simulink model "TestStructure"  (R2023b)
settings: Solver=FixedStepDiscrete  StartTime=0.0  StopTime=inf  FixedStep=SampleTime  RelTol=1e-3
InitFcn:
  | SampleTime = 0.001;
  | ButtonValue=0;
  | load("BusConfig.mat");
undefined symbols (not defined in the file): DiscIntNeverNeededParam
libraries: slrealtimeethercatlib x219, dspfdesign x28, dspstat3 x23, simulink x21, slpidlib x10, dspswit3 x8, commfilt2 x2, dspsigops x1
(part 4 of 8)

== system TestStructure/InterForceControlTask/AO3/Filter ==
  In : Inport
  Highpass Filter : dspfdesign/Highpass Filter  FilterType=IIR  DesignForMinimumOrder=on  FilterOrder=50  StopbandFrequency=0.015  PassbandFrequency=0.3  StopbandAttenuation=80  PassbandRipple=0.1  SampleRateMode=Specify on dialog  SampleRate=1000  SimulateUsing=Interpreted execution  roundingMode=Floor  coeffsDataTypeStr=fixdt(1,16)
  Highpass Filter1 : dspfdesign/Highpass Filter  FilterType=IIR  DesignForMinimumOrder=on  FilterOrder=50  StopbandFrequency=0.2  PassbandFrequency=0.3  StopbandAttenuation=60  PassbandRipple=1  SampleRateMode=Specify on dialog  SampleRate=1000  SimulateUsing=Code generation  roundingMode=Floor  coeffsDataTypeStr=fixdt(1,16)
  Lowpass Filter : dspfdesign/Lowpass Filter  FilterType=IIR  DesignForMinimumOrder=on  FilterOrder=50  PassbandFrequency=2.3  StopbandFrequency=4.3  PassbandRipple=0.1  StopbandAttenuation=80  SampleRateMode=Specify on dialog  SampleRate=1000  SimulateUsing=Interpreted execution  roundingMode=Floor  coeffsDataTypeStr=fixdt(1,16)
  Lowpass Filter1 : dspfdesign/Lowpass Filter  FilterType=IIR  DesignForMinimumOrder=on  FilterOrder=50  PassbandFrequency=6  StopbandFrequency=8  PassbandRipple=1  StopbandAttenuation=60  SampleRateMode=Specify on dialog  SampleRate=1000  SimulateUsing=Code generation  roundingMode=Floor  coeffsDataTypeStr=fixdt(1,16)
  Out : Outport
  wires:
  Highpass Filter1/1 -> Lowpass Filter1/1
  In/1 -> Highpass Filter/1
  Lowpass Filter/1 -> Out/1
  Highpass Filter/1 -> Lowpass Filter/1

== system TestStructure/InterForceControlTask/AO3/PhaseCorrection ==
  note: Subsystem
  Peaks : Inport
  Clock : Clock
  Constant3 : Constant
  Discrete-Time Integrator : DiscreteIntegrator  ExternalReset=rising  SampleTime=-1  ICPrevOutput=DiscIntNeverNeededParam  ICPrevScaledInput=DiscIntNeverNeededParam
  If : If  IfExpression=u1 == 1
  If Action Subsystem : Subsystem  TreatAsAtomicUnit=on
  If Action Subsystem1 : Subsystem  TreatAsAtomicUnit=on
  MATLAB Function : MATLAB Function  TreatAsAtomicUnit=on
  MATLAB Function1 : MATLAB Function  TreatAsAtomicUnit=on
  Merge : Merge
  Omega : Outport
  Phi_Corrected : Outport  Port=2
  wires:
  Clock/1 -> MATLAB Function1/2(t)
  MATLAB Function1/1(valid_peak) -> If/1
  Peaks/1 -> MATLAB Function1/1(raw_peak)
  If/1 -> If Action Subsystem/Action
  Discrete-Time Integrator/1 -> MATLAB Function/1(t_t_start)
  If/2 -> If Action Subsystem1/Action
  Merge/1 -> Discrete-Time Integrator/2, MATLAB Function/2(u)
  Constant3/1 -> Discrete-Time Integrator/1
  If Action Subsystem1/1(Out1) -> Merge/2
  If Action Subsystem/1(Out1) -> Merge/1
  MATLAB Function/1(Omega) -> Omega/1
  MATLAB Function/2(phi) -> Phi_Corrected/1

== system TestStructure/InterForceControlTask/AO3/Select ==
  P : Inport
  Phi : Inport  Port=2
  q : Inport  Port=3
  Abs : Abs  SaturateOnIntegerOverflow=off
  Add : Sum
  Add1 : Sum
  Bias1 : Bias  SaturateOnIntegerOverflow=off
  Bias2 : Bias  Bias=-0.001  SaturateOnIntegerOverflow=off
  Data Type Conversion : DataTypeConversion  OutDataTypeStr=double  SaturateOnIntegerOverflow=off  RndMeth=Floor
  Edge Detector : dspswit3/Edge Detector
  Gain1 : Gain  Gain=0.6
  Gain2 : Gain  OutDataTypeStr=Inherit: Same as input  ParamDataTypeStr=Inherit: Same as input
  Gain3 : Gain  Gain=0.1
  If : If  NumInputs=2  IfExpression=(u1 >= 10.5)|(u2 <= 1)
  If Action Subsystem : Subsystem  TreatAsAtomicUnit=on
  If Action Subsystem1 : Subsystem  TreatAsAtomicUnit=on
  MATLAB Function1 : MATLAB Function  TreatAsAtomicUnit=on
  Merge : Merge
  Merge1 : Merge
  Moving Average : dspstat3/Moving Average  Method=Sliding window  ForgettingFactorPort=off  SpecifyWindowLength=on  WindowLength=2000  OverlapLength=1999  AllowArbitraryInputLength=off  ForgettingFactor=0.9  SimulateUsing=Code generation
  Moving Average1 : dspstat3/Moving Average  Method=Sliding window  ForgettingFactorPort=off  SpecifyWindowLength=on  WindowLength=2000  OverlapLength=1999  AllowArbitraryInputLength=off  ForgettingFactor=0.9  SimulateUsing=Code generation
  Saturation : Saturate  UpperLimit=inf  LowerLimit=0
  Phi_Out : Outport
  Phase0Event : Outport  Port=2
  wires:
  Bias1/1 -> If Action Subsystem/2(Phase0)
  If Action Subsystem/2(Phase0Event) -> Merge1/2
  If Action Subsystem1/2(Out2) -> Merge1/1
  If Action Subsystem/1(Phi_Out) -> Merge/2
  Add1/1 -> If/2
  Data Type Conversion/1 -> Gain2/1
  Gain3/1 -> Add1/1
  Moving Average1/1 -> Add1/2
  q/1 -> MATLAB Function1/1(u)
  MATLAB Function1/1(y) -> Abs/1
  Abs/1 -> Moving Average1/1, Gain3/1
  Merge1/1 -> Phase0Event/1
  Merge/1 -> Phi_Out/1
  If/2 -> If Action Subsystem/Action
  Add/1 -> If/1
  If/1 -> If Action Subsystem1/Action
  Gain2/1 -> Bias1/1
  Moving Average/1 -> Add/2
  Saturation/1 -> Edge Detector/1
  Edge Detector/1 -> Data Type Conversion/1
  Phi/1 -> If Action Subsystem/1(Phi), Bias2/1
  Bias2/1 -> Saturation/1
  P/1 -> Moving Average/1, Gain1/1
  Gain1/1 -> Add/1
  If Action Subsystem1/1(Out1) -> Merge/1

== system TestStructure/InterForceControlTask/AO3/Subsystem ==
  q : Inport
  f : Inport  Port=2
  Add : Sum  Inputs=++++
  Gain1 : Gain  Gain=1/(2*pi)
  Gain2 : Gain  Gain=1/(2*pi)
  Subsystem : Subsystem
      settings: PortSchema="{\"entries\":[{\"content\":{\"sides\":[{\"content\":{\"connectorIds\":[\"In1\",\"In2\",\"In3\"]},\"type\":\"ConnectorPlacement.EquallySpacedRectSide\",\"uuid\":\"fcadf485-1c54-4f3f-872d-ec2f9b882f19\"},{\"content\":{\"connectorIds\":[\"Out1\",\"Out2\",\"Out3\",\"Out4\"],\"side\":\"RIGHT\"},\"type\":\"ConnectorPlacement.EquallySpacedRectSide\",\"uuid\":\"c1591880-cfe2-422f-a22e-44609bf238b6\"},{\"content\":{\"connectorIds\":[\"In4\"],\"side\":\"TOP\"},\"type\":\"ConnectorPlacement.EquallySpacedRectSide\",\"uuid\":\"5e5eda86-5041-4cab-91db-6a7c0e12be81\"}]},\"type\":\"ConnectorPlacement.EquallySpacedConnector\",\"uuid\":\"19c16159-ed31-430a-9428-452ee8c26aba\"}],\"packageUris\":[\"http://schema.mathworks.com/mf0/Connector/R2020b\"],\"version\":\"1.0\"}"
  Subsystem1 : Subsystem
  Subsystem2 : Subsystem
      settings: PortSchema="{\"entries\":[{\"content\":{\"sides\":[{\"content\":{\"connectorIds\":[\"In1\",\"In2\",\"In3\"]},\"type\":\"ConnectorPlacement.EquallySpacedRectSide\",\"uuid\":\"8ec379b7-ae46-4480-a29c-58696021cca5\"},{\"content\":{\"connectorIds\":[\"Out1\",\"Out2\",\"Out3\"],\"side\":\"RIGHT\"},\"type\":\"ConnectorPlacement.EquallySpacedRectSide\",\"uuid\":\"cda231b2-17f5-4d36-92f5-7ce39ba724b7\"},{\"content\":{\"connectorIds\":[],\"side\":\"TOP\"},\"type\":\"ConnectorPlacement.EquallySpacedRectSide\",\"uuid\":\"4db6421b-b56f-479d-b059-30db4d04c79c\"},{\"content\":{\"connectorIds\":[\"Out4\"],\"side\":\"BOTTOM\"},\"type\":\"ConnectorPlacement.EquallySpacedRectSide\",\"uuid\":\"ff0451e3-8881-4680-9eeb-8c81f572143a\"}]},\"type\":\"ConnectorPlacement.EquallySpacedConnector\",\"uuid\":\"26cfb436-360b-4c37-a6b2-80fa044f0317\"}],\"packageUris\":[\"http://schema.mathworks.com/mf0/Connector/R2020b\"],\"version\":\"1.0\"}"
  Subsystem3 : Subsystem
  Subsystem5 : Subsystem
  x : Outport
  Omega : Outport  Port=2
  Phi : Outport  Port=3
  P : Outport  Port=4
  wires:
  f/1 -> Subsystem/4(f)
  Subsystem/2(Omega) -> Subsystem1/3(Omega), Subsystem3/2(Omega), Subsystem5/3(Omega), Gain1/1
  Subsystem2/4(P) -> P/1
  Subsystem5/1(x) -> Add/4
  Subsystem3/1(x) -> Add/3
  Subsystem2/3(P(t)_Phi) -> Subsystem/3(P(t)_Phi), Subsystem1/2(P(t)_Phi), Subsystem3/3(P(t)_Phi), Subsystem5/2(P(t)_Phi)
  Subsystem1/1(x) -> Add/2
  Subsystem2/2(P(t)_Omega) -> Subsystem/2(P(t)_Omega)
  Subsystem2/1(P(t)_x) -> Subsystem/1(P(t)_x), Subsystem1/1(P(t)_x), Subsystem3/1(P(t)_x), Subsystem5/1(P(t)_x)
  Gain1/1 -> Omega/1
  Subsystem/3(Phi) -> Gain2/1
  Subsystem/1(x) -> Add/1
  Gain2/1 -> Phi/1
  Add/1 -> x/1, Subsystem2/2(X(t))
  q/1 -> Subsystem2/1(T(t))

== system TestStructure/InterForceControlTask/AO3/Subsystem1 ==
  note: Subsystem
  note: ZeroCrossFinder
  q : Inport
  Constant3 : Constant
  Discrete Derivative : simulink/Discrete/Discrete Derivative  gainval=1.0  ICPrevScaledInput=0.0  OutMin=[]  OutMax=[]  OutDataType=fixdt(1, 16)  OutScaling=2^-10  DoSatur=off
  Discrete-Time Integrator : DiscreteIntegrator  ExternalReset=rising  SampleTime=-1  ICPrevOutput=DiscIntNeverNeededParam  ICPrevScaledInput=DiscIntNeverNeededParam
  If : If  IfExpression=u1 == 1
  If Action Subsystem : Subsystem  TreatAsAtomicUnit=on
  If Action Subsystem1 : Subsystem  TreatAsAtomicUnit=on
  If Action Subsystem2 : Subsystem  TreatAsAtomicUnit=on
  If Action Subsystem3 : Subsystem  TreatAsAtomicUnit=on
  If1 : If
  Math Function : Math  Operator=reciprocal
  Memory : Memory
  Merge : Merge
  Merge1 : Merge
  Moving Maximum : dspstat3/Moving Maximum  SpecifyWindowLength=on  WindowLength=3  SimulateUsing=Code generation
  Moving Minimum : dspstat3/Moving Minimum  SpecifyWindowLength=on  WindowLength=3  SimulateUsing=Code generation
  Sign : Signum
  Triggered Subsystem : Subsystem  TreatAsAtomicUnit=on
  f : Outport
  Peak : Outport  Port=2
  wires:
  Discrete Derivative/1 -> Sign/1
  Sign/1 -> If1/1
  If1/1 -> If Action Subsystem2/Action
  If1/2 -> If Action Subsystem3/Action
  If Action Subsystem2/1(Out1) -> Merge1/1
  If Action Subsystem3/1(Out1) -> Merge1/2
  q/1 -> Discrete Derivative/1, Moving Minimum/1, If Action Subsystem2/1(q), Moving Maximum/1, If Action Subsystem3/1(q)
  Moving Minimum/1 -> If Action Subsystem2/2(WindowMin)
  Moving Maximum/1 -> If Action Subsystem3/2(WindowMax)
  Discrete-Time Integrator/1 -> Memory/1
  Merge1/1 -> Peak/1, If/1
  If/2 -> If Action Subsystem1/Action
  Merge/1 -> Triggered Subsystem/Trigger, Discrete-Time Integrator/2
  If/1 -> If Action Subsystem/Action
  Constant3/1 -> Discrete-Time Integrator/1
  If Action Subsystem1/1(Out1) -> Merge/2
  If Action Subsystem/1(Out1) -> Merge/1
  Memory/1 -> Triggered Subsystem/1(In1)
  Math Function/1 -> f/1
  Triggered Subsystem/1(t-t_start) -> Math Function/1

== system TestStructure/InterForceControlTask/DMP/ParamLatch ==
  In1 : Inport
  Enable : EnablePort
  Out1 : Outport
  wires:
  In1/1 -> Out1/1

== system TestStructure/InterForceControlTask/DMP/PhaseTimer ==
  t_now : Inport
  Trigger : TriggerPort  VariantControl=(inherit)
  Add : Sum  Inputs=+-
  UD_tlast : UnitDelay  SampleTime=-1  HasFrameUpgradeWarning=on
  ChunkSize : Outport
  wires:
  UD_tlast/1 -> Add/2
  Add/1 -> ChunkSize/1  "t_prev"
  t_now/1 -> Add/1, UD_tlast/1  "t_now"

== system TestStructure/InterForceControlTask/DMP/Subsystem ==
  ratio : Inport
  trig_in : Inport  Port=2
  t_prev : Inport  Port=3
  T_base_default : Inport  Port=4
  tau : Inport  Port=5
  BaseNormalizedStep : Product  Inputs=*/
  BasePeriodFloor : MinMax  Function=max  Inputs=2
  DelaySamplesFromPrev : MATLAB Function  TreatAsAtomicUnit=on
  EventDelay : MATLAB Function  TreatAsAtomicUnit=on
  Gain1 : Gain  Gain=1/1000
  MinBasePeriod : Constant  Value=0.005
  PhiOmega_DelayRebuild : MATLAB Function  TreatAsAtomicUnit=on
  dt1 : Constant  Value=0.001
  Phase0Event_Delay : Outport
  Phi_Delay : Outport  Port=2
  Omega_Delay : Outport  Port=3
  wires:
  DelaySamplesFromPrev/1(N) -> EventDelay/2(N)
  ratio/1 -> DelaySamplesFromPrev/2(ratio)
  t_prev/1 -> DelaySamplesFromPrev/1(t_prev), BasePeriodFloor/1
  trig_in/1 -> EventDelay/1(trig_in)
  dt1/1 -> DelaySamplesFromPrev/3(dt), BaseNormalizedStep/1, PhiOmega_DelayRebuild/2(dt_sec)
  PhiOmega_DelayRebuild/2(omega_delay) -> Gain1/1
  EventDelay/1(out) -> Phase0Event_Delay/1, PhiOmega_DelayRebuild/1(event_delay)
  PhiOmega_DelayRebuild/1(phi_delay) -> Phi_Delay/1
  tau/1 -> EventDelay/3(tau)
  MinBasePeriod/1 -> BasePeriodFloor/2
  BasePeriodFloor/1 -> BaseNormalizedStep/2
  BaseNormalizedStep/1 -> Omega_Delay/1
  T_base_default/1 -> PhiOmega_DelayRebuild/3(T_base_default)

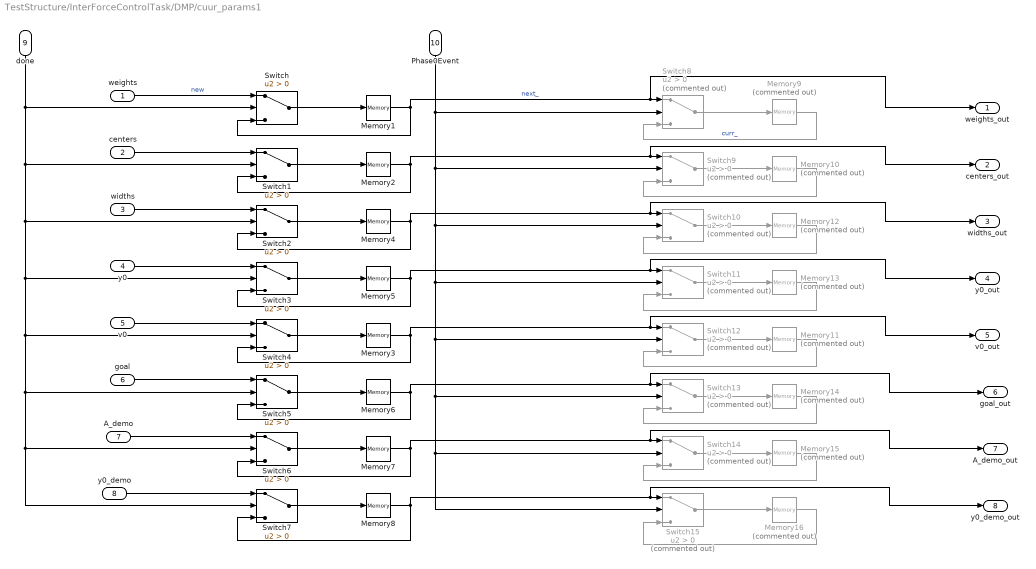
== system TestStructure/InterForceControlTask/DMP/cuur_params1 ==
  weights : Inport
  centers : Inport  Port=2
  widths : Inport  Port=3
  y0 : Inport  Port=4
  v0 : Inport  Port=5
  goal : Inport  Port=6
  A_demo : Inport  Port=7
  y0_demo : Inport  Port=8
  done : Inport  Port=9
  Phase0Event : Inport  Port=10
  Memory{1..2,4,7} (4 alike) : Memory  InitialCondition=1
  Memory{9..10,12,15} (4 alike) : Memory  Commented=on  InitialCondition=1
  Memory{11,13..14,16} (4 alike) : Memory  Commented=on
  Memory{3,5..6,8} (4 alike) : Memory
  Switch{,1..7} (8 alike) : Switch  Criteria=u2 > Threshold  SaturateOnIntegerOverflow=off  InputSameDT=off
  Switch{8..15} (8 alike) : Switch  Commented=on  Criteria=u2 > Threshold  SaturateOnIntegerOverflow=off  InputSameDT=off
  weights_out : Outport
  centers_out : Outport  Port=2
  widths_out : Outport  Port=3
  y0_out : Outport  Port=4
  v0_out : Outport  Port=5
  goal_out : Outport  Port=6
  A_demo_out : Outport  Port=7
  y0_demo_out : Outport  Port=8
  wires:
  Memory10/1 -> Switch9/3
  Switch8/1 -> Memory9/1
  Switch9/1 -> Memory10/1
  Memory1/1 -> Switch8/1, weights_out/1, Switch/3  "next_"
  Switch11/1 -> Memory13/1
  Memory7/1 -> Switch6/3, Switch14/1, A_demo_out/1
  Switch14/1 -> Memory15/1
  Switch10/1 -> Memory12/1
  Switch12/1 -> Memory11/1
  Switch13/1 -> Memory14/1
  Switch15/1 -> Memory16/1
  Phase0Event/1 -> Switch15/2, Switch14/2, Switch13/2, Switch12/2, Switch11/2, Switch10/2, Switch9/2, Switch8/2
  Memory11/1 -> Switch12/3
  Memory6/1 -> Switch5/3, Switch13/1, goal_out/1
  Memory16/1 -> Switch15/3
  Memory15/1 -> Switch14/3
  Memory14/1 -> Switch13/3
  Memory4/1 -> Switch2/3, Switch10/1, widths_out/1
  Memory5/1 -> Switch3/3, Switch11/1, y0_out/1
  Memory12/1 -> Switch10/3
  Memory3/1 -> Switch4/3, Switch12/1, v0_out/1
  Memory2/1 -> Switch1/3, Switch9/1, centers_out/1
  Memory9/1 -> Switch8/3  "curr_"
  Memory13/1 -> Switch11/3
  Memory8/1 -> Switch7/3, Switch15/1, y0_demo_out/1
  weights/1 -> Switch/1  "new"
  centers/1 -> Switch1/1
  widths/1 -> Switch2/1
  y0/1 -> Switch3/1
  v0/1 -> Switch4/1
  goal/1 -> Switch5/1
  A_demo/1 -> Switch6/1
  y0_demo/1 -> Switch7/1
  done/1 -> Switch/2, Switch1/2, Switch2/2, Switch3/2, Switch4/2, Switch5/2, Switch6/2, Switch7/2
  Switch/1 -> Memory1/1
  Switch1/1 -> Memory2/1
  Switch2/1 -> Memory4/1
  Switch3/1 -> Memory5/1
  Switch7/1 -> Memory8/1
  Switch6/1 -> Memory7/1
  Switch5/1 -> Memory6/1
  Switch4/1 -> Memory3/1

== system TestStructure/InterForceControlTask/TorqueController/Filter1 ==
  In : Inport
  Highpass Filter : dspfdesign/Highpass Filter  FilterType=IIR  DesignForMinimumOrder=on  FilterOrder=50  StopbandFrequency=0.015  PassbandFrequency=0.3  StopbandAttenuation=80  PassbandRipple=0.1  SampleRateMode=Specify on dialog  SampleRate=1000  SimulateUsing=Interpreted execution  roundingMode=Floor  coeffsDataTypeStr=fixdt(1,16)
  Highpass Filter1 : dspfdesign/Highpass Filter  FilterType=IIR  DesignForMinimumOrder=on  FilterOrder=50  StopbandFrequency=0.29  PassbandFrequency=0.3  StopbandAttenuation=60  PassbandRipple=1  SampleRateMode=Specify on dialog  SampleRate=1000  SimulateUsing=Code generation  roundingMode=Floor  coeffsDataTypeStr=fixdt(1,16)
  Lowpass Filter : dspfdesign/Lowpass Filter  FilterType=IIR  DesignForMinimumOrder=on  FilterOrder=50  PassbandFrequency=2.3  StopbandFrequency=4.3  PassbandRipple=0.1  StopbandAttenuation=80  SampleRateMode=Specify on dialog  SampleRate=1000  SimulateUsing=Interpreted execution  roundingMode=Floor  coeffsDataTypeStr=fixdt(1,16)
  Lowpass Filter1 : dspfdesign/Lowpass Filter  FilterType=IIR  DesignForMinimumOrder=on  FilterOrder=50  PassbandFrequency=6  StopbandFrequency=8  PassbandRipple=1  StopbandAttenuation=60  SampleRateMode=Specify on dialog  SampleRate=1000  SimulateUsing=Code generation  roundingMode=Floor  coeffsDataTypeStr=fixdt(1,16)
  Out : Outport
  wires:
  Highpass Filter1/1 -> Lowpass Filter1/1
  In/1 -> Highpass Filter1/1
  Lowpass Filter1/1 -> Out/1
  Highpass Filter/1 -> Lowpass Filter/1

== system TestStructure/InterForceControlTask/TorqueController/If Action Subsystem1 ==
  Action Port : ActionPort  ActionPortLabel=if((u1 >= u2))
  ActivityValue : Constant
  activity_gain : Outport
  wires:
  ActivityValue/1 -> activity_gain/1

== system TestStructure/InterForceControlTask/TorqueController/If Action Subsystem_activity_on ==
  Action Port : ActionPort  ActionPortLabel=else
  ActivityValue : Constant  Value=0
  activity_gain : Outport
  wires:
  ActivityValue/1 -> activity_gain/1

== system TestStructure/InterForceControlTask/TorqueController/Subsystem2 ==
  note: ZeroCrossFinder
  q : Inport
  Abs : Abs  Commented=on  SaturateOnIntegerOverflow=off
  Buffer : Buffer  Commented=on  N=30  V=29  OutputFrames=off
  Buffer Function : MATLAB Function  TreatAsAtomicUnit=on
  Constant1 : Constant
  Discrete Derivative : simulink/Discrete/Discrete Derivative  gainval=1.0  ICPrevScaledInput=0.0  OutMin=[]  OutMax=[]  OutDataType=fixdt(1, 16)  OutScaling=2^-10  DoSatur=off
  Function-Call Subsystem : Subsystem  TreatAsAtomicUnit=on
  Function-Call Subsystem1 : Subsystem  TreatAsAtomicUnit=on
  Function-Call Subsystem2 : Subsystem  TreatAsAtomicUnit=on
  Gain : Gain  Gain=0.4
  Gain2 : Gain  Gain=-1
  If Action Subsystem2 : Subsystem  TreatAsAtomicUnit=on
  If Action Subsystem3 : Subsystem  TreatAsAtomicUnit=on
  If1 : If  IfExpression=(u1 > -0.02)&(u1<0.02)
  If2 : If  NumInputs=2  IfExpression=(u1 > u2)  ElseIfExpressions=(u1< -u2)
  MATLAB Function : MATLAB Function  Commented=on  TreatAsAtomicUnit=on
  Merge1 : Merge
  Merge2 : Merge
  Merge3 : Merge  Inputs=3
  Moving Maximum : dspstat3/Moving Maximum  SpecifyWindowLength=on  WindowLength=2000  SimulateUsing=Code generation
  Product : Product
  Switch : Switch  Criteria=u2 > Threshold  SaturateOnIntegerOverflow=off  InputSameDT=off
  Windowed Integrator : commfilt2/Windowed Integrator  Commented=on  integperiod=600  roundingMode=Floor  overflowMode=off  coeffDataTypeStr=Inherit: Same word length as input  coeffMin=[]  coeffMax=[]  coeffLastDataTypeStr=Inherit: Same word length as input  accumDataTypeStr=Inherit: Same as product output  accumLastDataTypeStr=Inherit: Same as product output  outputDataTypeStr=Inherit: Same as accumulator  outputMin=[]  outputMax=[]  outputLastDataTypeStr=Inherit: Same as accumulator
  threadhold : Constant  Value=0.1
  Peak : Outport  OutputWhenDisabled=reset  InitialOutput=[0]
  wires:
  q/1 -> Discrete Derivative/1, Buffer Function/1(u)
  If Action Subsystem3/1(Out1) -> Merge1/2
  If Action Subsystem2/1(Out1) -> Merge1/1
  If1/2 -> If Action Subsystem3/Action
  If1/1 -> If Action Subsystem2/Action
  Discrete Derivative/1 -> If1/1
  Buffer Function/1(y) -> If Action Subsystem2/1(WindowMin)
  If Action Subsystem2/2(Out2) -> Merge2/1
  If Action Subsystem3/2(Out2) -> Merge2/2
  Merge2/1 -> Product/2
  If Action Subsystem2/3(y) -> Product/1
  Function-Call Subsystem/1(Out1) -> Merge3/1  "1"
  Function-Call Subsystem1/1(Out1) -> Merge3/3  "0"
  If2/1 -> Function-Call Subsystem/Action
  If2/3 -> Function-Call Subsystem1/Action
  Function-Call Subsystem2/1(Out1) -> Merge3/2  "-1"
  If2/2 -> Function-Call Subsystem2/Action
  Moving Maximum/1 -> Gain/1
  Gain/1 -> If2/2
  Switch/1 -> If2/1, Moving Maximum/1
  Gain2/1 -> Switch/3
  Constant1/1 -> Switch/2
  Abs/1 -> Windowed Integrator/1
  Windowed Integrator/1 -> MATLAB Function/1(u)
  Product/1 -> Gain2/1, Switch/1, Abs/1
  MATLAB Function/1(y) -> ?
  threadhold/1 -> If Action Subsystem2/2(threadhold)
  Merge3/1 -> Peak/1

== system TestStructure/InterForceControlTask/TorqueController/TorqueManager ==
  activity_enable : Inport
  valid_peak : Inport  Port=2
  target_torque : Inport  Port=3
  MO_drop ? steps : Gain  Gain=0  ParamDataTypeStr=double  OutDataTypeStr=double
  MO_step ramp ? per 5 : Gain  ParamDataTypeStr=double  OutDataTypeStr=double
  activity <= 0 : simulink/Logic and Bit Operations/Compare To Constant  relop=<=  const=0  OutDataTypeStr=boolean
  activity falling edge : Logic  AllPortsSameDT=off  OutDataTypeStr=boolean
  base_gain 0..1 : Saturate  UpperLimit=1  LowerLimit=0  OutDataTypeStr=double
  count + step : Sum  Inputs=++-  OutDataTypeStr=double  AccumDataTypeStr=double
  if activity : simulink/Logic and Bit Operations/Compare To Constant  relop=>  const=0  OutDataTypeStr=boolean
  prev_activity : UnitDelay  SampleTime=-1  HasFrameUpgradeWarning=on
  prev_activity > 0 : simulink/Logic and Bit Operations/Compare To Constant  relop=>  const=0  OutDataTypeStr=boolean
  prev_peak : UnitDelay  SampleTime=-1  HasFrameUpgradeWarning=on
  prev_peak <= 0.5 : simulink/Logic and Bit Operations/Compare To Constant  relop=<=  const=0.5  OutDataTypeStr=boolean
  rising valid step : Logic  Inputs=3  AllPortsSameDT=off  OutDataTypeStr=boolean
  step_count 0..5 : Saturate  UpperLimit=5  LowerLimit=0  OutDataTypeStr=double
  step_count memory : UnitDelay  InitialCondition=0.0  SampleTime=-1  HasFrameUpgradeWarning=on
  torque gate : Product  Inputs=**  OutDataTypeStr=double
  valid_peak > 0.5 : simulink/Logic and Bit Operations/Compare To Constant  relop=>  const=0.5  OutDataTypeStr=boolean
  actual_torque : Outport
  current_gain : Outport  Port=2
  wires:
  valid_peak/1 -> valid_peak > 0.5/1, prev_peak/1
  prev_peak/1 -> prev_peak <= 0.5/1
  valid_peak > 0.5/1 -> rising valid step/1
  prev_peak <= 0.5/1 -> rising valid step/2
  activity_enable/1 -> if activity/1, activity <= 0/1, prev_activity/1
  if activity/1 -> rising valid step/3
  step_count memory/1 -> count + step/1
  rising valid step/1 -> count + step/2
  count + step/1 -> step_count 0..5/1
  MO_step ramp ? per 5/1 -> base_gain 0..1/1
  base_gain 0..1/1 -> current_gain/1, torque gate/2
  target_torque/1 -> torque gate/1
  torque gate/1 -> actual_torque/1
  prev_activity > 0/1 -> activity falling edge/2
  prev_activity/1 -> prev_activity > 0/1
  activity <= 0/1 -> activity falling edge/1
  activity falling edge/1 -> MO_drop ? steps/1
  MO_drop ? steps/1 -> count + step/3
  step_count 0..5/1 -> step_count memory/1, MO_step ramp ? per 5/1

== system TestStructure/InterForceControlTask/TorqueController2/Filter ==
  q : Inport
  Highpass Filter : dspfdesign/Highpass Filter  FilterType=IIR  DesignForMinimumOrder=on  FilterOrder=50  StopbandFrequency=0.015  PassbandFrequency=0.3  StopbandAttenuation=80  PassbandRipple=0.1  SampleRateMode=Specify on dialog  SampleRate=1000  SimulateUsing=Interpreted execution  roundingMode=Floor  coeffsDataTypeStr=fixdt(1,16)
  Highpass Filter1 : dspfdesign/Highpass Filter  FilterType=IIR  DesignForMinimumOrder=on  FilterOrder=50  StopbandFrequency=0.2  PassbandFrequency=0.3  StopbandAttenuation=60  PassbandRipple=1  SampleRateMode=Specify on dialog  SampleRate=1000  SimulateUsing=Code generation  roundingMode=Floor  coeffsDataTypeStr=fixdt(1,16)
  Lowpass Filter : dspfdesign/Lowpass Filter  FilterType=IIR  DesignForMinimumOrder=on  FilterOrder=50  PassbandFrequency=2.3  StopbandFrequency=4.3  PassbandRipple=0.1  StopbandAttenuation=80  SampleRateMode=Specify on dialog  SampleRate=1000  SimulateUsing=Interpreted execution  roundingMode=Floor  coeffsDataTypeStr=fixdt(1,16)
  Lowpass Filter1 : dspfdesign/Lowpass Filter  FilterType=IIR  DesignForMinimumOrder=on  FilterOrder=50  PassbandFrequency=6  StopbandFrequency=8  PassbandRipple=1  StopbandAttenuation=60  SampleRateMode=Specify on dialog  SampleRate=1000  SimulateUsing=Code generation  roundingMode=Floor  coeffsDataTypeStr=fixdt(1,16)
  Out : Outport
  wires:
  Highpass Filter1/1 -> Lowpass Filter1/1
  q/1 -> Highpass Filter/1
  Lowpass Filter/1 -> Out/1
  Highpass Filter/1 -> Lowpass Filter/1

== system TestStructure/InterForceControlTask/TorqueController2/ZeroCrossFinder_Right ==
  note: ZeroCrossFinder
  U : Inport
  Discrete Derivative1 : simulink/Discrete/Discrete Derivative  gainval=1.0  ICPrevScaledInput=0.0  OutMin=[]  OutMax=[]  OutDataType=fixdt(1, 16)  OutScaling=2^-10  DoSatur=off
  If Action Subsystem1 : Subsystem  TreatAsAtomicUnit=on
  If Action Subsystem4 : Subsystem  TreatAsAtomicUnit=on
  If2 : If  IfExpression=(u1 > -0.005)|(u1<0.005)
  Merge2 : Merge
  Moving Minimum1 : dspstat3/Moving Minimum  SpecifyWindowLength=on  WindowLength=3  SimulateUsing=Code generation
  peak_right : Outport
  wires:
  U/1 -> Discrete Derivative1/1, Moving Minimum1/1
  If Action Subsystem1/1(Out1) -> Merge2/1
  If Action Subsystem4/1(Out1) -> Merge2/2
  If2/1 -> If Action Subsystem1/Action
  Moving Minimum1/1 -> If Action Subsystem1/1(WindowMin)
  If2/2 -> If Action Subsystem4/Action
  Discrete Derivative1/1 -> If2/1
  Merge2/1 -> peak_right/1

== system TestStructure/InterForceControlTask/Torque_Guard/LimitProtect ==
  LeftHipMotorTorque : Inport
  RightHipMotorTorque : Inport  Port=2
  <WhichFoot> : Inport  Port=3
  <LeftHipMotorActuralPosition> : Inport  Port=4
  <RightHipMotorActuralPosition> : Inport  Port=5
  Gain : Gain  Gain=-1
  Gain1 : Gain  Gain=-1
  Logical Operator : Logic  Operator=NOT  AllPortsSameDT=off  OutDataTypeStr=boolean
  Logical Operator1 : Logic  Operator=NOT  AllPortsSameDT=off  OutDataTypeStr=boolean
  Logical Operator2 : Logic  Operator=OR  AllPortsSameDT=off  OutDataTypeStr=boolean
  Logical Operator3 : Logic  Operator=OR  AllPortsSameDT=off  OutDataTypeStr=boolean
  Logical Operator4 : Logic  Operator=OR  AllPortsSameDT=off  OutDataTypeStr=boolean
  Relay : Relay  OnSwitchValue=90  OffSwitchValue=30
  Relay1 : Relay  OnSwitchValue=90  OffSwitchValue=30
  SafeTorque : Constant  Value=20
  Switch{,1..4} (5 alike) : Switch  Criteria=u2 > Threshold  SaturateOnIntegerOverflow=off  InputSameDT=off
  LeftHipMotorTorque_safe : Outport
  RightHipMotorTorque_safe : Outport  Port=2
  wires:
  Switch3/1 -> LeftHipMotorTorque_safe/1
  <WhichFoot>/1 -> Switch/2, Logical Operator1/1, Logical Operator3/1
  <LeftHipMotorActuralPosition>/1 -> Switch/3, Gain1/1
  <RightHipMotorActuralPosition>/1 -> Gain/1, Switch/1
  RightHipMotorTorque/1 -> Switch2/3, Switch1/1
  Switch2/1 -> RightHipMotorTorque_safe/1
  LeftHipMotorTorque/1 -> Switch4/1, Switch3/3
  Switch1/1 -> Switch2/1
  SafeTorque/1 -> Switch1/3, Switch4/3
  Switch4/1 -> Switch3/1
  Logical Operator/1 -> Switch1/2, Switch4/2
  Logical Operator1/1 -> Logical Operator4/2
  Gain/1 -> Relay/1
  Gain1/1 -> Relay1/1
  Relay/1 -> Logical Operator2/1
  Relay1/1 -> Logical Operator2/2
  Logical Operator2/1 -> Logical Operator/1, Logical Operator4/1, Logical Operator3/2
  Logical Operator3/1 -> Switch2/2
  Logical Operator4/1 -> Switch3/2

== system TestStructure/InterForceControlTask/Torque_Guard/MinimumTauGate ==
  tau_e : Inport
  In2 : Inport  Port=2
  In3 : Inport  Port=3
  DirectTquInSwinging : ManualSwitch
  MO_AffectedLegdefault : Constant  Value=0
  Switch2 : Switch  Criteria=u2 > Threshold  SaturateOnIntegerOverflow=off  InputSameDT=off
  ToGiveTquInStanding? : ManualSwitch  CurrentSetting=0
  Out1 : Outport
  wires:
  In2/1 -> ToGiveTquInStanding?/2
  tau_e/1 -> Switch2/3, DirectTquInSwinging/2
  In3/1 -> Switch2/2
  MO_AffectedLegdefault/1 -> ToGiveTquInStanding?/1
  ToGiveTquInStanding?/1 -> Switch2/1
  DirectTquInSwinging/1 -> Out1/1
  Switch2/1 -> DirectTquInSwinging/1

== system TestStructure/InterForceControlTask/Torque_Guard/SwingTauRelease ==
  tau_e : Inport
  In2 : Inport  Port=2
  In3 : Inport  Port=3
  Switch2 : Switch  Criteria=u2 > Threshold  SaturateOnIntegerOverflow=off  InputSameDT=off
  Out1 : Outport
  wires:
  In3/1 -> Switch2/2
  tau_e/1 -> Switch2/3
  Switch2/1 -> Out1/1
  In2/1 -> Switch2/1

== system TestStructure/Robot/MotorPositonInit1/If Action Subsystem5 ==
  In1 : Inport
  Action Port : ActionPort  ActionPortLabel=if((u1 > 3.6))
  Out1 : Outport
  wires:
  In1/1 -> Out1/1

== system TestStructure/Robot/MotorPositonInit1/If Action Subsystem6 ==
  In1 : Inport
  Action Port : ActionPort  ActionPortLabel=else
  Out1 : Outport
  wires:
  In1/1 -> Out1/1

== system TestStructure/Robot/MotorPositonInit1/Subsystem ==
  MotorDesirePos : Inport
  MotorPos : Inport  Port=2
  MotorVel : Inport  Port=3
  Add : Sum
  Discrete PID Controller : slpidlib/PID Controller  Controller=PID  Form=Parallel  TimeDomain=Discrete-time  UseExternalTs=off  SampleTime=-1  IntegratorMethod=Forward Euler  FilterMethod=Forward Euler  ControllerParametersSource=internal  P=220  I=1  UseKiTs=off  D=2  N=100  UseFilter=on  TunerSelectOption=Transfer Function Based (PID Tuner App)  InitialConditionSource=internal  InitialConditionForIntegrator=0  InitialConditionForFilter=0  DifferentiatorICPrevScaledInput=0  ExternalReset=none  TrackingMode=off  Kt=1  LimitOutput=off  SatLimitsSource=internal  UpperSaturationLimit=inf  LowerSaturationLimit=-inf  LinearizeAsGain=off  AntiWindupMode=none  Kb=1  LimitIntegrator=off  UpperIntegratorSaturationLimit=inf  LowerIntegratorSaturationLimit=-inf  POutMin=[]  POutMax=[]  IOutMin=[]  IOutMax=[]  DOutMin=[]  DOutMax=[]  NOutMin=[]  NOutMax=[]  SumOutMin=[]  SumOutMax=[]  SaturationOutMin=[]  SaturationOutMax=[]  PParamMin=[]  PParamMax=[]  IParamMin=[]  IParamMax=[]  DParamMin=[]  DParamMax=[]  NParamMin=[]  NParamMax=[]  KbParamMin=[]  KbParamMax=[]  KtParamMin=[]  KtParamMax=[]  KbOutMin=[]  KbOutMax=[]  KtOutMin=[]  KtOutMax=[]  IntegratorOutMin=[]  IntegratorOutMax=[]  FilterOutMin=[]  FilterOutMax=[]  SumI1OutMin=[]  SumI1OutMax=[]  SumI2OutMin=[]  SumI2OutMax=[]  SumI3OutMin=[]  SumI3OutMax=[]  SumI4OutMin=[]  SumI4OutMax=[]  SumDOutMin=[]  SumDOutMax=[]  DifferentiatorOutMin=[]  DifferentiatorOutMax=[]  FilterDiffOutCoefMin=[]  FilterDiffOutCoefMax=[]  ReciprocalOutMin=[]  ReciprocalOutMax=[]  SumDenOutMin=[]  SumDenOutMax=[]  SumNumOutMin=[]  SumNumOutMax=[]  DivideOutMin=[]  DivideOutMax=[]  UdiffTsProdOutMin=[]  UdiffTsProdOutMax=[]  NTsProdOutMin=[]  NTsProdOutMax=[]  UintegralTsProdOutMin=[]  UintegralTsProdOutMax=[]  UngainTsProdOutMin=[]  UngainTsProdOutMax=[]  ClampingZeroOutDataTypeStr=Inherit: Inherit via back propagation  ClampingZeroOutMin=[]  ClampingZeroOutMax=[]  FilterDenConstantOutDataTypeStr=Inherit: Inherit via back propagation  FilterDenConstantOutMin=[]  FilterDenConstantOutMax=[]  PCopyOutDataTypeStr=Inherit: Inherit via back propagation  PCopyOutMin=[]  PCopyOutMax=[]  NCopyOutDataTypeStr=Inherit: Inherit via back propagation  NCopyOutMin=[]  NCopyOutMax=[]  IntegratorContinuousStateAttributes=''  IntegratorStateMustResolveToSignalObject=off  IntegratorRTWStateStorageClass=Auto  FilterContinuousStateAttributes=''  FilterStateMustResolveToSignalObject=off  FilterRTWStateStorageClass=Auto  ParallelPVariant=InternalParameters  IdealPVariant=Disabled  IVariant=InternalParameters  DVariant=InternalParameters  IntegratorVariant=Discrete  SatVariant=Disabled  AWVariant=Passthrough  PCopyVariant=Disabled  TRVariant=Disabled  FdbkBlocksVariant=Forward  IdealPFdbkVariant=Disabled  SatFdbkVariant=Disabled  DerivativeFilterVariant=ForwardEulerFilter  NVariant=InternalParameters  NCopyVariant=Disabled  FilterICVariant=InternalICsFilter  IntegratorICVariant=InternalICs  ExternalResetVariant=Disabled  TRSumVariant=Passthrough  SumFdbkVariant=Disabled  SumVariant=Sum_PID  TsampFilterVariant=InternalTs  TsampNgainVariant=Passthrough  TsampIntegralVariant=Passthrough  ExternalSaturationOutDataTypeStr=Inherit: Same as second input
      settings: LibrarySourceBlock=simulink/Discrete/Discrete PID Controller
  Discrete PID Controller1 : slpidlib/PID Controller  Controller=PD  Form=Parallel  TimeDomain=Discrete-time  UseExternalTs=off  SampleTime=-1  IntegratorMethod=Forward Euler  FilterMethod=Forward Euler  ControllerParametersSource=internal  P=0.0035  I=1  UseKiTs=off  D=0.00005  N=100  UseFilter=on  TunerSelectOption=Transfer Function Based (PID Tuner App)  InitialConditionSource=internal  InitialConditionForIntegrator=0  InitialConditionForFilter=0  DifferentiatorICPrevScaledInput=0  ExternalReset=none  TrackingMode=off  Kt=1  LimitOutput=on  SatLimitsSource=internal  UpperSaturationLimit=15  LowerSaturationLimit=-15  LinearizeAsGain=off  AntiWindupMode=none  Kb=1  LimitIntegrator=off  UpperIntegratorSaturationLimit=inf  LowerIntegratorSaturationLimit=-inf  POutMin=[]  POutMax=[]  IOutMin=[]  IOutMax=[]  DOutMin=[]  DOutMax=[]  NOutMin=[]  NOutMax=[]  SumOutMin=[]  SumOutMax=[]  SaturationOutMin=[]  SaturationOutMax=[]  PParamMin=[]  PParamMax=[]  IParamMin=[]  IParamMax=[]  DParamMin=[]  DParamMax=[]  NParamMin=[]  NParamMax=[]  KbParamMin=[]  KbParamMax=[]  KtParamMin=[]  KtParamMax=[]  KbOutMin=[]  KbOutMax=[]  KtOutMin=[]  KtOutMax=[]  IntegratorOutMin=[]  IntegratorOutMax=[]  FilterOutMin=[]  FilterOutMax=[]  SumI1OutMin=[]  SumI1OutMax=[]  SumI2OutMin=[]  SumI2OutMax=[]  SumI3OutMin=[]  SumI3OutMax=[]  SumI4OutMin=[]  SumI4OutMax=[]  SumDOutMin=[]  SumDOutMax=[]  DifferentiatorOutMin=[]  DifferentiatorOutMax=[]  FilterDiffOutCoefMin=[]  FilterDiffOutCoefMax=[]  ReciprocalOutMin=[]  ReciprocalOutMax=[]  SumDenOutMin=[]  SumDenOutMax=[]  SumNumOutMin=[]  SumNumOutMax=[]  DivideOutMin=[]  DivideOutMax=[]  UdiffTsProdOutMin=[]  UdiffTsProdOutMax=[]  NTsProdOutMin=[]  NTsProdOutMax=[]  UintegralTsProdOutMin=[]  UintegralTsProdOutMax=[]  UngainTsProdOutMin=[]  UngainTsProdOutMax=[]  ClampingZeroOutDataTypeStr=Inherit: Inherit via back propagation  ClampingZeroOutMin=[]  ClampingZeroOutMax=[]  FilterDenConstantOutDataTypeStr=Inherit: Inherit via back propagation  FilterDenConstantOutMin=[]  FilterDenConstantOutMax=[]  PCopyOutDataTypeStr=Inherit: Inherit via back propagation  PCopyOutMin=[]  PCopyOutMax=[]  NCopyOutDataTypeStr=Inherit: Inherit via back propagation  NCopyOutMin=[]  NCopyOutMax=[]  IntegratorContinuousStateAttributes=''  IntegratorStateMustResolveToSignalObject=off  IntegratorRTWStateStorageClass=Auto  FilterContinuousStateAttributes=''  FilterStateMustResolveToSignalObject=off  FilterRTWStateStorageClass=Auto  ParallelPVariant=InternalParameters  IdealPVariant=Disabled  IVariant=Disabled  DVariant=InternalParameters  IntegratorVariant=Disabled  SatVariant=Enabled  AWVariant=Disabled  PCopyVariant=Disabled  TRVariant=Disabled  FdbkBlocksVariant=Forward  IdealPFdbkVariant=Disabled  SatFdbkVariant=Disabled  DerivativeFilterVariant=ForwardEulerFilter  NVariant=InternalParameters  NCopyVariant=Disabled  FilterICVariant=InternalICsFilter  IntegratorICVariant=Disabled  ExternalResetVariant=Disabled  TRSumVariant=Passthrough  SumFdbkVariant=Disabled  SumVariant=Sum_PD  TsampFilterVariant=InternalTs  TsampNgainVariant=Passthrough  TsampIntegralVariant=Disabled_SignalSpec  ExternalSaturationOutDataTypeStr=Inherit: Same as second input
      settings: LibrarySourceBlock=simulink/Discrete/Discrete PID Controller
  Saturation2 : Saturate  UpperLimit=30  LowerLimit=-30
  Subtract : Sum  Inputs=+-
  Sum : Sum  Inputs=|+-
  Sum2 : Sum  Inputs=|+-
  MotorTorque : Outport
  wires:
  Discrete PID Controller1/1 -> MotorTorque/1
  Sum/1 -> Discrete PID Controller/1
  Sum2/1 -> Discrete PID Controller1/1
  MotorDesirePos/1 -> Sum/1
  MotorPos/1 -> Sum/2
  Saturation2/1 -> Add/2
  Add/1 -> Sum2/2
  Discrete PID Controller/1 -> Add/1, Subtract/2, Sum2/1
  MotorVel/1 -> Subtract/1
  Subtract/1 -> Saturation2/1

== system TestStructure/Robot/MotorPositonInit1/Subsystem1 ==
  MotorDesirePos : Inport
  MotorPos : Inport  Port=2
  MotorVel : Inport  Port=3
  Discrete PID Controller : slpidlib/PID Controller  Controller=PID  Form=Parallel  TimeDomain=Discrete-time  UseExternalTs=off  SampleTime=-1  IntegratorMethod=Forward Euler  FilterMethod=Forward Euler  ControllerParametersSource=internal  P=220  I=1  UseKiTs=off  D=2  N=100  UseFilter=on  TunerSelectOption=Transfer Function Based (PID Tuner App)  InitialConditionSource=internal  InitialConditionForIntegrator=0  InitialConditionForFilter=0  DifferentiatorICPrevScaledInput=0  ExternalReset=none  TrackingMode=off  Kt=1  LimitOutput=off  SatLimitsSource=internal  UpperSaturationLimit=inf  LowerSaturationLimit=-inf  LinearizeAsGain=off  AntiWindupMode=none  Kb=1  LimitIntegrator=off  UpperIntegratorSaturationLimit=inf  LowerIntegratorSaturationLimit=-inf  POutMin=[]  POutMax=[]  IOutMin=[]  IOutMax=[]  DOutMin=[]  DOutMax=[]  NOutMin=[]  NOutMax=[]  SumOutMin=[]  SumOutMax=[]  SaturationOutMin=[]  SaturationOutMax=[]  PParamMin=[]  PParamMax=[]  IParamMin=[]  IParamMax=[]  DParamMin=[]  DParamMax=[]  NParamMin=[]  NParamMax=[]  KbParamMin=[]  KbParamMax=[]  KtParamMin=[]  KtParamMax=[]  KbOutMin=[]  KbOutMax=[]  KtOutMin=[]  KtOutMax=[]  IntegratorOutMin=[]  IntegratorOutMax=[]  FilterOutMin=[]  FilterOutMax=[]  SumI1OutMin=[]  SumI1OutMax=[]  SumI2OutMin=[]  SumI2OutMax=[]  SumI3OutMin=[]  SumI3OutMax=[]  SumI4OutMin=[]  SumI4OutMax=[]  SumDOutMin=[]  SumDOutMax=[]  DifferentiatorOutMin=[]  DifferentiatorOutMax=[]  FilterDiffOutCoefMin=[]  FilterDiffOutCoefMax=[]  ReciprocalOutMin=[]  ReciprocalOutMax=[]  SumDenOutMin=[]  SumDenOutMax=[]  SumNumOutMin=[]  SumNumOutMax=[]  DivideOutMin=[]  DivideOutMax=[]  UdiffTsProdOutMin=[]  UdiffTsProdOutMax=[]  NTsProdOutMin=[]  NTsProdOutMax=[]  UintegralTsProdOutMin=[]  UintegralTsProdOutMax=[]  UngainTsProdOutMin=[]  UngainTsProdOutMax=[]  ClampingZeroOutDataTypeStr=Inherit: Inherit via back propagation  ClampingZeroOutMin=[]  ClampingZeroOutMax=[]  FilterDenConstantOutDataTypeStr=Inherit: Inherit via back propagation  FilterDenConstantOutMin=[]  FilterDenConstantOutMax=[]  PCopyOutDataTypeStr=Inherit: Inherit via back propagation  PCopyOutMin=[]  PCopyOutMax=[]  NCopyOutDataTypeStr=Inherit: Inherit via back propagation  NCopyOutMin=[]  NCopyOutMax=[]  IntegratorContinuousStateAttributes=''  IntegratorStateMustResolveToSignalObject=off  IntegratorRTWStateStorageClass=Auto  FilterContinuousStateAttributes=''  FilterStateMustResolveToSignalObject=off  FilterRTWStateStorageClass=Auto  ParallelPVariant=InternalParameters  IdealPVariant=Disabled  IVariant=InternalParameters  DVariant=InternalParameters  IntegratorVariant=Discrete  SatVariant=Disabled  AWVariant=Passthrough  PCopyVariant=Disabled  TRVariant=Disabled  FdbkBlocksVariant=Forward  IdealPFdbkVariant=Disabled  SatFdbkVariant=Disabled  DerivativeFilterVariant=ForwardEulerFilter  NVariant=InternalParameters  NCopyVariant=Disabled  FilterICVariant=InternalICsFilter  IntegratorICVariant=InternalICs  ExternalResetVariant=Disabled  TRSumVariant=Passthrough  SumFdbkVariant=Disabled  SumVariant=Sum_PID  TsampFilterVariant=InternalTs  TsampNgainVariant=Passthrough  TsampIntegralVariant=Disabled_SignalSpec  ExternalSaturationOutDataTypeStr=Inherit: Same as second input
      settings: LibrarySourceBlock=simulink/Discrete/Discrete PID Controller
  Discrete PID Controller1 : slpidlib/PID Controller  Controller=PD  Form=Parallel  TimeDomain=Discrete-time  UseExternalTs=off  SampleTime=-1  IntegratorMethod=Forward Euler  FilterMethod=Forward Euler  ControllerParametersSource=internal  P=0.0035  I=1  UseKiTs=off  D=0.00005  N=100  UseFilter=on  TunerSelectOption=Transfer Function Based (PID Tuner App)  InitialConditionSource=internal  InitialConditionForIntegrator=0  InitialConditionForFilter=0  DifferentiatorICPrevScaledInput=0  ExternalReset=none  TrackingMode=off  Kt=1  LimitOutput=on  SatLimitsSource=internal  UpperSaturationLimit=15  LowerSaturationLimit=-15  LinearizeAsGain=off  AntiWindupMode=none  Kb=1  LimitIntegrator=off  UpperIntegratorSaturationLimit=inf  LowerIntegratorSaturationLimit=-inf  POutMin=[]  POutMax=[]  IOutMin=[]  IOutMax=[]  DOutMin=[]  DOutMax=[]  NOutMin=[]  NOutMax=[]  SumOutMin=[]  SumOutMax=[]  SaturationOutMin=[]  SaturationOutMax=[]  PParamMin=[]  PParamMax=[]  IParamMin=[]  IParamMax=[]  DParamMin=[]  DParamMax=[]  NParamMin=[]  NParamMax=[]  KbParamMin=[]  KbParamMax=[]  KtParamMin=[]  KtParamMax=[]  KbOutMin=[]  KbOutMax=[]  KtOutMin=[]  KtOutMax=[]  IntegratorOutMin=[]  IntegratorOutMax=[]  FilterOutMin=[]  FilterOutMax=[]  SumI1OutMin=[]  SumI1OutMax=[]  SumI2OutMin=[]  SumI2OutMax=[]  SumI3OutMin=[]  SumI3OutMax=[]  SumI4OutMin=[]  SumI4OutMax=[]  SumDOutMin=[]  SumDOutMax=[]  DifferentiatorOutMin=[]  DifferentiatorOutMax=[]  FilterDiffOutCoefMin=[]  FilterDiffOutCoefMax=[]  ReciprocalOutMin=[]  ReciprocalOutMax=[]  SumDenOutMin=[]  SumDenOutMax=[]  SumNumOutMin=[]  SumNumOutMax=[]  DivideOutMin=[]  DivideOutMax=[]  UdiffTsProdOutMin=[]  UdiffTsProdOutMax=[]  NTsProdOutMin=[]  NTsProdOutMax=[]  UintegralTsProdOutMin=[]  UintegralTsProdOutMax=[]  UngainTsProdOutMin=[]  UngainTsProdOutMax=[]  ClampingZeroOutDataTypeStr=Inherit: Inherit via back propagation  ClampingZeroOutMin=[]  ClampingZeroOutMax=[]  FilterDenConstantOutDataTypeStr=Inherit: Inherit via back propagation  FilterDenConstantOutMin=[]  FilterDenConstantOutMax=[]  PCopyOutDataTypeStr=Inherit: Inherit via back propagation  PCopyOutMin=[]  PCopyOutMax=[]  NCopyOutDataTypeStr=Inherit: Inherit via back propagation  NCopyOutMin=[]  NCopyOutMax=[]  IntegratorContinuousStateAttributes=''  IntegratorStateMustResolveToSignalObject=off  IntegratorRTWStateStorageClass=Auto  FilterContinuousStateAttributes=''  FilterStateMustResolveToSignalObject=off  FilterRTWStateStorageClass=Auto  ParallelPVariant=InternalParameters  IdealPVariant=Disabled  IVariant=Disabled  DVariant=InternalParameters  IntegratorVariant=Disabled  SatVariant=Enabled  AWVariant=Disabled  PCopyVariant=Disabled  TRVariant=Disabled  FdbkBlocksVariant=Forward  IdealPFdbkVariant=Disabled  SatFdbkVariant=Disabled  DerivativeFilterVariant=ForwardEulerFilter  NVariant=InternalParameters  NCopyVariant=Disabled  FilterICVariant=InternalICsFilter  IntegratorICVariant=Disabled  ExternalResetVariant=Disabled  TRSumVariant=Passthrough  SumFdbkVariant=Disabled  SumVariant=Sum_PD  TsampFilterVariant=InternalTs  TsampNgainVariant=Passthrough  TsampIntegralVariant=Disabled_SignalSpec  ExternalSaturationOutDataTypeStr=Inherit: Same as second input
      settings: LibrarySourceBlock=simulink/Discrete/Discrete PID Controller
  Saturation1 : Saturate  UpperLimit=60  LowerLimit=-60
  Sum : Sum  Inputs=|+-
  Sum1 : Sum  Inputs=|+-
  MotorTorque : Outport
  wires:
  Discrete PID Controller1/1 -> MotorTorque/1
  Sum/1 -> Discrete PID Controller/1
  Saturation1/1 -> Sum1/2
  Discrete PID Controller/1 -> Sum1/1
  Sum1/1 -> Discrete PID Controller1/1
  MotorDesirePos/1 -> Sum/1
  MotorVel/1 -> Saturation1/1
  MotorPos/1 -> Sum/2

== system TestStructure/Robot/MotorPositonInit1/Subsystem2 ==
  MotorDesirePos : Inport
  MotorPos : Inport  Port=2
  MotorVel : Inport  Port=3
  Discrete PID Controller : slpidlib/PID Controller  Controller=PID  Form=Parallel  TimeDomain=Discrete-time  UseExternalTs=off  SampleTime=-1  IntegratorMethod=Forward Euler  FilterMethod=Forward Euler  ControllerParametersSource=internal  P=220  I=1  UseKiTs=off  D=2  N=100  UseFilter=on  TunerSelectOption=Transfer Function Based (PID Tuner App)  InitialConditionSource=internal  InitialConditionForIntegrator=0  InitialConditionForFilter=0  DifferentiatorICPrevScaledInput=0  ExternalReset=none  TrackingMode=off  Kt=1  LimitOutput=off  SatLimitsSource=internal  UpperSaturationLimit=inf  LowerSaturationLimit=-inf  LinearizeAsGain=off  AntiWindupMode=none  Kb=1  LimitIntegrator=off  UpperIntegratorSaturationLimit=inf  LowerIntegratorSaturationLimit=-inf  POutMin=[]  POutMax=[]  IOutMin=[]  IOutMax=[]  DOutMin=[]  DOutMax=[]  NOutMin=[]  NOutMax=[]  SumOutMin=[]  SumOutMax=[]  SaturationOutMin=[]  SaturationOutMax=[]  PParamMin=[]  PParamMax=[]  IParamMin=[]  IParamMax=[]  DParamMin=[]  DParamMax=[]  NParamMin=[]  NParamMax=[]  KbParamMin=[]  KbParamMax=[]  KtParamMin=[]  KtParamMax=[]  KbOutMin=[]  KbOutMax=[]  KtOutMin=[]  KtOutMax=[]  IntegratorOutMin=[]  IntegratorOutMax=[]  FilterOutMin=[]  FilterOutMax=[]  SumI1OutMin=[]  SumI1OutMax=[]  SumI2OutMin=[]  SumI2OutMax=[]  SumI3OutMin=[]  SumI3OutMax=[]  SumI4OutMin=[]  SumI4OutMax=[]  SumDOutMin=[]  SumDOutMax=[]  DifferentiatorOutMin=[]  DifferentiatorOutMax=[]  FilterDiffOutCoefMin=[]  FilterDiffOutCoefMax=[]  ReciprocalOutMin=[]  ReciprocalOutMax=[]  SumDenOutMin=[]  SumDenOutMax=[]  SumNumOutMin=[]  SumNumOutMax=[]  DivideOutMin=[]  DivideOutMax=[]  UdiffTsProdOutMin=[]  UdiffTsProdOutMax=[]  NTsProdOutMin=[]  NTsProdOutMax=[]  UintegralTsProdOutMin=[]  UintegralTsProdOutMax=[]  UngainTsProdOutMin=[]  UngainTsProdOutMax=[]  ClampingZeroOutDataTypeStr=Inherit: Inherit via back propagation  ClampingZeroOutMin=[]  ClampingZeroOutMax=[]  FilterDenConstantOutDataTypeStr=Inherit: Inherit via back propagation  FilterDenConstantOutMin=[]  FilterDenConstantOutMax=[]  PCopyOutDataTypeStr=Inherit: Inherit via back propagation  PCopyOutMin=[]  PCopyOutMax=[]  NCopyOutDataTypeStr=Inherit: Inherit via back propagation  NCopyOutMin=[]  NCopyOutMax=[]  IntegratorContinuousStateAttributes=''  IntegratorStateMustResolveToSignalObject=off  IntegratorRTWStateStorageClass=Auto  FilterContinuousStateAttributes=''  FilterStateMustResolveToSignalObject=off  FilterRTWStateStorageClass=Auto  ParallelPVariant=InternalParameters  IdealPVariant=Disabled  IVariant=InternalParameters  DVariant=InternalParameters  IntegratorVariant=Discrete  SatVariant=Disabled  AWVariant=Passthrough  PCopyVariant=Disabled  TRVariant=Disabled  FdbkBlocksVariant=Forward  IdealPFdbkVariant=Disabled  SatFdbkVariant=Disabled  DerivativeFilterVariant=ForwardEulerFilter  NVariant=InternalParameters  NCopyVariant=Disabled  FilterICVariant=InternalICsFilter  IntegratorICVariant=InternalICs  ExternalResetVariant=Disabled  TRSumVariant=Passthrough  SumFdbkVariant=Disabled  SumVariant=Sum_PID  TsampFilterVariant=InternalTs  TsampNgainVariant=Passthrough  TsampIntegralVariant=Disabled_SignalSpec  ExternalSaturationOutDataTypeStr=Inherit: Same as second input
      settings: LibrarySourceBlock=simulink/Discrete/Discrete PID Controller
  Discrete PID Controller1 : slpidlib/PID Controller  Controller=PD  Form=Parallel  TimeDomain=Discrete-time  UseExternalTs=off  SampleTime=-1  IntegratorMethod=Forward Euler  FilterMethod=Forward Euler  ControllerParametersSource=internal  P=0.0035  I=1  UseKiTs=off  D=0.00005  N=100  UseFilter=on  TunerSelectOption=Transfer Function Based (PID Tuner App)  InitialConditionSource=internal  InitialConditionForIntegrator=0  InitialConditionForFilter=0  DifferentiatorICPrevScaledInput=0  ExternalReset=none  TrackingMode=off  Kt=1  LimitOutput=on  SatLimitsSource=internal  UpperSaturationLimit=15  LowerSaturationLimit=-15  LinearizeAsGain=off  AntiWindupMode=none  Kb=1  LimitIntegrator=off  UpperIntegratorSaturationLimit=inf  LowerIntegratorSaturationLimit=-inf  POutMin=[]  POutMax=[]  IOutMin=[]  IOutMax=[]  DOutMin=[]  DOutMax=[]  NOutMin=[]  NOutMax=[]  SumOutMin=[]  SumOutMax=[]  SaturationOutMin=[]  SaturationOutMax=[]  PParamMin=[]  PParamMax=[]  IParamMin=[]  IParamMax=[]  DParamMin=[]  DParamMax=[]  NParamMin=[]  NParamMax=[]  KbParamMin=[]  KbParamMax=[]  KtParamMin=[]  KtParamMax=[]  KbOutMin=[]  KbOutMax=[]  KtOutMin=[]  KtOutMax=[]  IntegratorOutMin=[]  IntegratorOutMax=[]  FilterOutMin=[]  FilterOutMax=[]  SumI1OutMin=[]  SumI1OutMax=[]  SumI2OutMin=[]  SumI2OutMax=[]  SumI3OutMin=[]  SumI3OutMax=[]  SumI4OutMin=[]  SumI4OutMax=[]  SumDOutMin=[]  SumDOutMax=[]  DifferentiatorOutMin=[]  DifferentiatorOutMax=[]  FilterDiffOutCoefMin=[]  FilterDiffOutCoefMax=[]  ReciprocalOutMin=[]  ReciprocalOutMax=[]  SumDenOutMin=[]  SumDenOutMax=[]  SumNumOutMin=[]  SumNumOutMax=[]  DivideOutMin=[]  DivideOutMax=[]  UdiffTsProdOutMin=[]  UdiffTsProdOutMax=[]  NTsProdOutMin=[]  NTsProdOutMax=[]  UintegralTsProdOutMin=[]  UintegralTsProdOutMax=[]  UngainTsProdOutMin=[]  UngainTsProdOutMax=[]  ClampingZeroOutDataTypeStr=Inherit: Inherit via back propagation  ClampingZeroOutMin=[]  ClampingZeroOutMax=[]  FilterDenConstantOutDataTypeStr=Inherit: Inherit via back propagation  FilterDenConstantOutMin=[]  FilterDenConstantOutMax=[]  PCopyOutDataTypeStr=Inherit: Inherit via back propagation  PCopyOutMin=[]  PCopyOutMax=[]  NCopyOutDataTypeStr=Inherit: Inherit via back propagation  NCopyOutMin=[]  NCopyOutMax=[]  IntegratorContinuousStateAttributes=''  IntegratorStateMustResolveToSignalObject=off  IntegratorRTWStateStorageClass=Auto  FilterContinuousStateAttributes=''  FilterStateMustResolveToSignalObject=off  FilterRTWStateStorageClass=Auto  ParallelPVariant=InternalParameters  IdealPVariant=Disabled  IVariant=Disabled  DVariant=InternalParameters  IntegratorVariant=Disabled  SatVariant=Enabled  AWVariant=Disabled  PCopyVariant=Disabled  TRVariant=Disabled  FdbkBlocksVariant=Forward  IdealPFdbkVariant=Disabled  SatFdbkVariant=Disabled  DerivativeFilterVariant=ForwardEulerFilter  NVariant=InternalParameters  NCopyVariant=Disabled  FilterICVariant=InternalICsFilter  IntegratorICVariant=Disabled  ExternalResetVariant=Disabled  TRSumVariant=Passthrough  SumFdbkVariant=Disabled  SumVariant=Sum_PD  TsampFilterVariant=InternalTs  TsampNgainVariant=Passthrough  TsampIntegralVariant=Disabled_SignalSpec  ExternalSaturationOutDataTypeStr=Inherit: Same as second input
      settings: LibrarySourceBlock=simulink/Discrete/Discrete PID Controller
  Saturation1 : Saturate  UpperLimit=60  LowerLimit=-60
  Sum : Sum  Inputs=|+-
  Sum1 : Sum  Inputs=|+-
  MotorTorque : Outport
  wires:
  Discrete PID Controller1/1 -> MotorTorque/1
  Sum/1 -> Discrete PID Controller/1
  Saturation1/1 -> Sum1/2
  Discrete PID Controller/1 -> Sum1/1
  Sum1/1 -> Discrete PID Controller1/1
  MotorDesirePos/1 -> Sum/1
  MotorVel/1 -> Saturation1/1
  MotorPos/1 -> Sum/2
